simulink model "limited_bit_width_sum_enob"  (R2013b)
settings: Solver=VariableStepDiscrete  StartTime=0.0  StopTime=StopTime  RelTol=1e-3
values from neighbouring files (symbols this model uses):
  a2 = a(2)    [design_2ord_sc_sigma_delta_adc_20211008.m]    (also in run_limited_bit_width_sum.m; run_limited_bit_width_sum_enob.m; run_tst1.m)
  amp = umax    [design_2ord_sc_sigma_delta_adc_20211008.m]    (also in run_limited_bit_width_sum.m; run_limited_bit_width_sum_enob.m = 0.8; run_tst1.m = 0.01)
  b1 = b(1)    [design_2ord_sc_sigma_delta_adc_20211008.m]    (also in run_limited_bit_width_sum.m; run_limited_bit_width_sum_enob.m; run_tst1.m)
  c1 = c(1)    [design_2ord_sc_sigma_delta_adc_20211008.m]    (also in run_limited_bit_width_sum.m; run_limited_bit_width_sum_enob.m; run_tst1.m)
  den = 2^(cic_order*log(osr)/log(2))    [design_2ord_sc_sigma_delta_adc_20211008.m]    (also in run_limited_bit_width_sum.m; run_limited_bit_width_sum_enob.m; run_tst1.m)
  fin = fs*7/128/osr    (= 0.213623046875)    [design_2ord_sc_sigma_delta_adc_20211008.m]    (also in run_limited_bit_width_sum.m = 54.6875; run_limited_bit_width_sum_enob.m; run_tst1.m = 54.6875)
  fs = 256e3    (= 256000)    [design_2ord_sc_sigma_delta_adc_20211008.m]    (also in run_limited_bit_width_sum.m; run_limited_bit_width_sum_enob.m; run_tst1.m)
  osr = 2^16    (= 65536)    [cal_c1_20211015.m]    (also in design_2ord_sc_sigma_delta_adc_20211008.m; run_limited_bit_width_sum.m = 256; run_limited_bit_width_sum_enob.m; run_tst1.m = 256)
  vos = 10e-3    (= 0.01)    [design_2ord_sc_sigma_delta_adc_20211008.m]    (also in run_limited_bit_width_sum.m; run_limited_bit_width_sum_enob.m)
  width_comb1 = 25    [design_2ord_sc_sigma_delta_adc_20211008.m]    (also in run_limited_bit_width_sum.m = width_comb1 - 1; run_limited_bit_width_sum_enob.m = width_comb1 + 1)
  width_comb2 = 20    [design_2ord_sc_sigma_delta_adc_20211008.m]    (also in run_limited_bit_width_sum.m = width_comb2 - 1; run_limited_bit_width_sum_enob.m = width_comb2 + 1)
  width_comb3 = 19    [design_2ord_sc_sigma_delta_adc_20211008.m]    (also in run_limited_bit_width_sum.m = width_comb3 - 1; run_limited_bit_width_sum_enob.m = width_comb3 + 1)
  width_int1 = 49    [design_2ord_sc_sigma_delta_adc_20211008.m]    (also in run_limited_bit_width_sum.m = width_int1 - 1; run_limited_bit_width_sum_enob.m = width_int1 + 1)
  width_int2 = 38    [design_2ord_sc_sigma_delta_adc_20211008.m]    (also in run_limited_bit_width_sum.m = width_int2 - 1; run_limited_bit_width_sum_enob.m = width_int2 + 1)
  width_int3 = 26    [design_2ord_sc_sigma_delta_adc_20211008.m]    (also in run_limited_bit_width_sum.m = width_int3 - 1; run_limited_bit_width_sum_enob.m = width_int3 + 1)
settings Model: Creator=eric  LastModifiedBy=eric

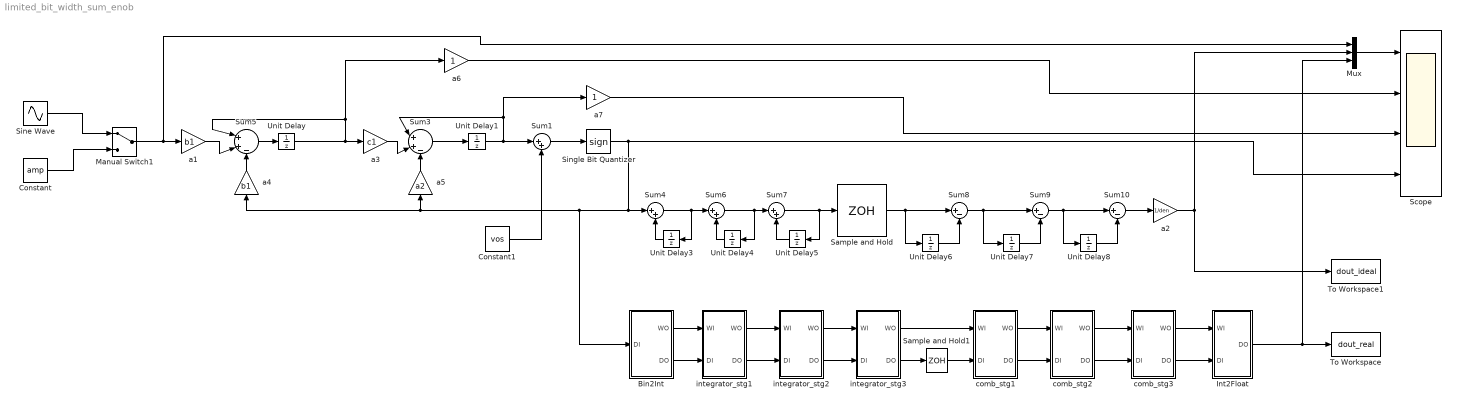
== system limited_bit_width_sum_enob ==
  Bin2Int : Subsystem
  Constant : Constant  Value=amp  SampleTime=1/fs
  Constant1 : Constant  Value=vos  SampleTime=1/fs
  Int2Float : Subsystem
  Manual Switch1 : ManualSwitch
  Mux : Mux  Inputs=3
  Sample and Hold : ZeroOrderHold  SampleTime=osr/fs
  Sample and Hold1 : ZeroOrderHold  SampleTime=osr/fs
  Scope : Scope  NumInputPorts=4
      settings: TimeRange=0.09  YMin=0.00999~-0.2~-0.2~-1.5  YMax=0.01001~0.6~0.2~1.5  MaxDataPoints=20000
  Sine Wave : Sin  Amplitude=amp  Frequency=2*pi*fin  SampleTime=1/fs
  Single Bit Quantizer : Signum  SampleTime=1/fs
  Sum{1,4,6..7} (4 alike) : Sum  Inputs=|++  AccumDataTypeStr=double  SampleTime=1/fs
  Sum10 : Sum  Inputs=|+-  AccumDataTypeStr=double  SampleTime=osr/fs
  Sum3 : Sum  Inputs=|++-  AccumDataTypeStr=double  SampleTime=1/fs
  Sum5 : Sum  Inputs=|++-  AccumDataTypeStr=double  SampleTime=1/fs
  Sum8 : Sum  Inputs=|+-  AccumDataTypeStr=double  SampleTime=osr/fs
  Sum9 : Sum  Inputs=|+-  AccumDataTypeStr=double  SampleTime=osr/fs
  To Workspace : ToWorkspace  VariableName=dout_real  SampleTime=osr/fs  SaveFormat=Timeseries
  To Workspace1 : ToWorkspace  VariableName=dout_ideal  SampleTime=osr/fs  SaveFormat=Timeseries
  Unit Delay{,1,3..5} (5 alike) : UnitDelay  SampleTime=1/fs
  Unit Delay6 : UnitDelay  SampleTime=osr/fs
  Unit Delay7 : UnitDelay  SampleTime=osr/fs
  Unit Delay8 : UnitDelay  SampleTime=osr/fs
  a1 : Gain  Gain=b1  SampleTime=1/fs
  a2 : Gain  Gain=1/den  SampleTime=osr/fs
  a3 : Gain  Gain=c1  SampleTime=1/fs
  a4 : Gain  Gain=b1  SampleTime=1/fs
  a5 : Gain  Gain=a2  SampleTime=1/fs
  a6 : Gain  SampleTime=1/fs
  a7 : Gain  SampleTime=1/fs
  comb_stg1 : Subsystem
  comb_stg2 : Subsystem
  comb_stg3 : Subsystem
  integrator_stg1 : Subsystem
  integrator_stg2 : Subsystem
  integrator_stg3 : Subsystem
  wires:
  Sum3/1 -> Unit Delay1/1
  Sum5/1 -> Unit Delay/1
  Unit Delay3/1 -> Sum4/2
  Sum4/1 -> Sum6/1, Unit Delay3/1
  Unit Delay4/1 -> Sum6/2
  Sum6/1 -> Unit Delay4/1, Sum7/1
  Unit Delay5/1 -> Sum7/2
  Sum7/1 -> Unit Delay5/1, Sample and Hold/1
  Sample and Hold/1 -> Unit Delay6/1, Sum8/1
  Unit Delay6/1 -> Sum8/2
  Unit Delay7/1 -> Sum9/2
  Sum8/1 -> Unit Delay7/1, Sum9/1
  Sum9/1 -> Unit Delay8/1, Sum10/1
  Unit Delay8/1 -> Sum10/2
  Sum10/1 -> a2/1
  a2/1 -> To Workspace1/1, Mux/2
  Manual Switch1/1 -> Mux/1, a1/1
  Sine Wave/1 -> Manual Switch1/1
  Constant/1 -> Manual Switch1/2
  Mux/1 -> Scope/1
  a4/1 -> Sum5/3
  a1/1 -> Sum5/2
  Unit Delay/1 -> a6/1, Sum5/1, a3/1
  a5/1 -> Sum3/3
  a3/1 -> Sum3/2
  Unit Delay1/1 -> Sum1/1, a7/1, Sum3/1
  a7/1 -> Scope/3
  a6/1 -> Scope/2
  Sum1/1 -> Single Bit Quantizer/1
  Constant1/1 -> Sum1/2
  integrator_stg1/1(WO) -> integrator_stg2/1(WI)
  integrator_stg1/2(DO) -> integrator_stg2/2(DI)
  integrator_stg2/1(WO) -> integrator_stg3/1(WI)
  integrator_stg2/2(DO) -> integrator_stg3/2(DI)
  comb_stg1/2(DO) -> comb_stg2/2(DI)
  comb_stg1/1(WO) -> comb_stg2/1(WI)
  comb_stg2/1(WO) -> comb_stg3/1(WI)
  comb_stg2/2(DO) -> comb_stg3/2(DI)
  integrator_stg3/1(WO) -> comb_stg1/1(WI)
  integrator_stg3/2(DO) -> Sample and Hold1/1
  Sample and Hold1/1 -> comb_stg1/2(DI)
  comb_stg3/1(WO) -> Int2Float/1(WI)
  comb_stg3/2(DO) -> Int2Float/2(DI)
  Int2Float/1(DO) -> To Workspace/1, Mux/3
  Single Bit Quantizer/1 -> Bin2Int/1(DI), a5/1, a4/1, Sum4/1, Scope/4
  Bin2Int/1(WO) -> integrator_stg1/1(WI)
  Bin2Int/2(DO) -> integrator_stg1/2(DI)

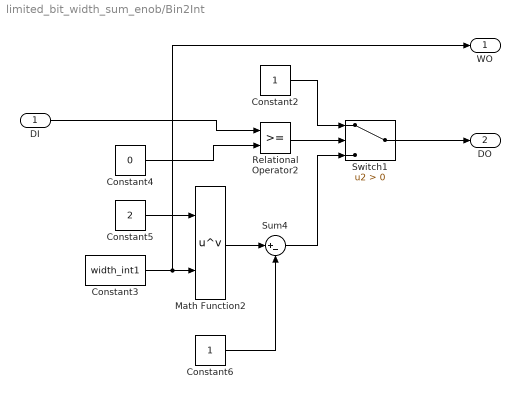
== system limited_bit_width_sum_enob/Bin2Int ==
  DI : Inport
  Constant2 : Constant
  Constant3 : Constant  Value=width_int1
  Constant4 : Constant  Value=0
  Constant5 : Constant  Value=2
  Constant6 : Constant
  Math Function2 : Math  Operator=pow  SampleTime=1/fs  SaturateOnIntegerOverflow=on
  Relational Operator2 : RelationalOperator  OutDataTypeStr=boolean  SampleTime=1/fs
  Sum4 : Sum  Inputs=|+-  SampleTime=1/fs
  Switch1 : Switch  Criteria=u2 > Threshold  SampleTime=1/fs
  WO : Outport
  DO : Outport  Port=2
  wires:
  Math Function2/1 -> Sum4/1
  Constant3/1 -> WO/1, Math Function2/2
  DI/1 -> Relational Operator2/1
  Switch1/1 -> DO/1
  Constant6/1 -> Sum4/2
  Relational Operator2/1 -> Switch1/2
  Constant2/1 -> Switch1/1
  Constant4/1 -> Relational Operator2/2
  Constant5/1 -> Math Function2/1
  Sum4/1 -> Switch1/3

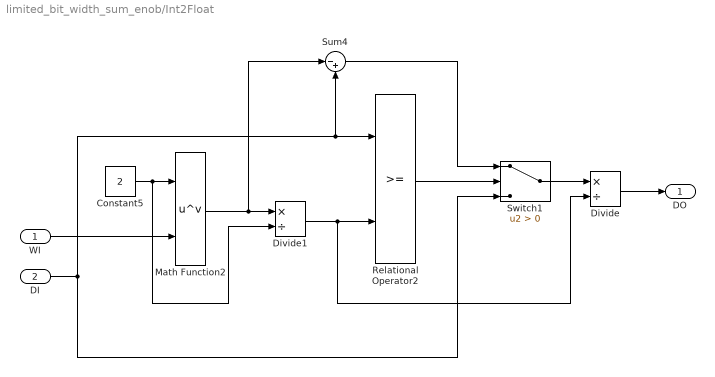
== system limited_bit_width_sum_enob/Int2Float ==
  WI : Inport
  DI : Inport  Port=2
  Constant5 : Constant  Value=2
  Divide : Product  Inputs=*/  SampleTime=1/fs
  Divide1 : Product  Inputs=*/  SampleTime=1/fs
  Math Function2 : Math  Operator=pow  SampleTime=1/fs  SaturateOnIntegerOverflow=on
  Relational Operator2 : RelationalOperator  OutDataTypeStr=boolean  SampleTime=1/fs
  Sum4 : Sum  Inputs=|-+  SampleTime=1/fs
  Switch1 : Switch  Criteria=u2 > Threshold  SampleTime=1/fs
  DO : Outport
  wires:
  Switch1/1 -> Divide/1
  Divide/1 -> DO/1
  Relational Operator2/1 -> Switch1/2
  Math Function2/1 -> Divide1/1, Sum4/1
  Sum4/1 -> Switch1/1
  Constant5/1 -> Divide1/2, Math Function2/1
  DI/1 -> Relational Operator2/1, Sum4/2, Switch1/3
  WI/1 -> Math Function2/2
  Divide1/1 -> Divide/2, Relational Operator2/2

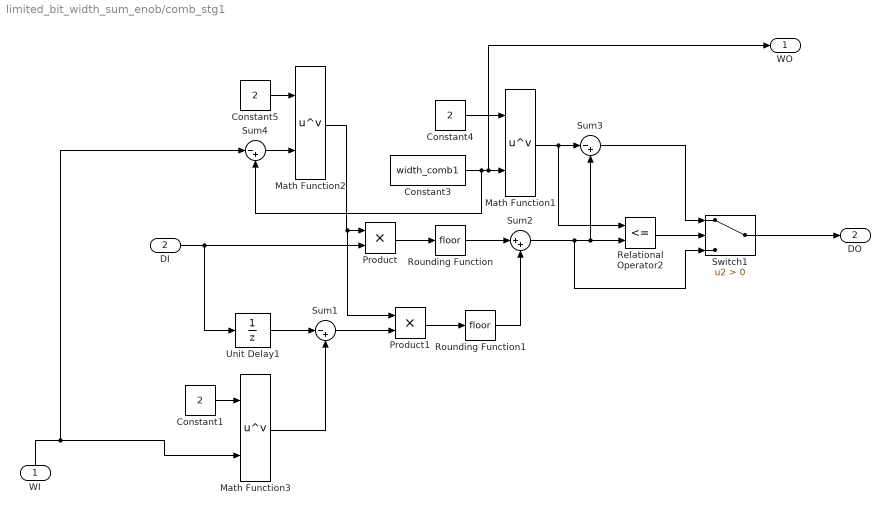
== system limited_bit_width_sum_enob/comb_stg1 ==
  WI : Inport
  DI : Inport  Port=2
  Constant1 : Constant  Value=2
  Constant3 : Constant  Value=width_comb1
  Constant4 : Constant  Value=2
  Constant5 : Constant  Value=2
  Math Function1 : Math  Operator=pow  SampleTime=1/fs  SaturateOnIntegerOverflow=on
  Math Function2 : Math  Operator=pow  SampleTime=1/fs  SaturateOnIntegerOverflow=on
  Math Function3 : Math  Operator=pow  SampleTime=1/fs  SaturateOnIntegerOverflow=on
  Product : Product  SampleTime=1/fs
  Product1 : Product  SampleTime=1/fs
  Relational Operator2 : RelationalOperator  Operator=<=  OutDataTypeStr=boolean  SampleTime=1/fs
  Rounding Function : Rounding  SampleTime=1/fs
  Rounding Function1 : Rounding  SampleTime=1/fs
  Sum1 : Sum  Inputs=|-+  SampleTime=1/fs
  Sum2 : Sum  Inputs=|++  SampleTime=1/fs
  Sum3 : Sum  Inputs=|-+  SampleTime=1/fs
  Sum4 : Sum  Inputs=|-+  SampleTime=1/fs
  Switch1 : Switch  Criteria=u2 > Threshold  SampleTime=1/fs
  Unit Delay1 : UnitDelay  SampleTime=osr/fs
  WO : Outport
  DO : Outport  Port=2
  wires:
  Sum4/1 -> Math Function2/2
  Constant5/1 -> Math Function2/1
  Rounding Function/1 -> Sum2/1
  Math Function2/1 -> Product1/1, Product/1
  Math Function1/1 -> Relational Operator2/1, Sum3/1
  Relational Operator2/1 -> Switch1/2
  Sum3/1 -> Switch1/1
  Sum2/1 -> Relational Operator2/2, Sum3/2, Switch1/3
  Product/1 -> Rounding Function/1
  Constant4/1 -> Math Function1/1
  WI/1 -> Math Function3/2, Sum4/1
  DI/1 -> Unit Delay1/1, Product/2
  Switch1/1 -> DO/1
  Constant1/1 -> Math Function3/1
  Constant3/1 -> Sum4/2, WO/1, Math Function1/2
  Unit Delay1/1 -> Sum1/1
  Math Function3/1 -> Sum1/2
  Rounding Function1/1 -> Sum2/2
  Product1/1 -> Rounding Function1/1
  Sum1/1 -> Product1/2

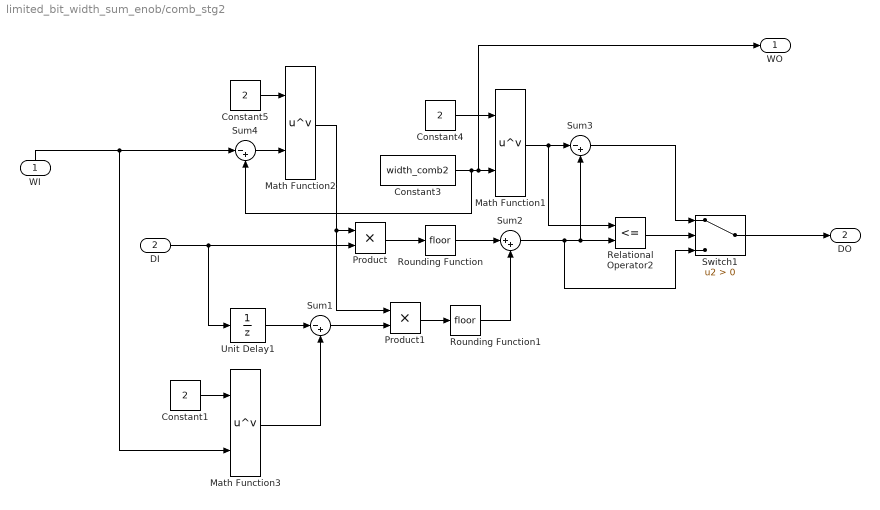
== system limited_bit_width_sum_enob/comb_stg2 ==
  WI : Inport
  DI : Inport  Port=2
  Constant1 : Constant  Value=2
  Constant3 : Constant  Value=width_comb2
  Constant4 : Constant  Value=2
  Constant5 : Constant  Value=2
  Math Function1 : Math  Operator=pow  SampleTime=1/fs  SaturateOnIntegerOverflow=on
  Math Function2 : Math  Operator=pow  SampleTime=1/fs  SaturateOnIntegerOverflow=on
  Math Function3 : Math  Operator=pow  SampleTime=1/fs  SaturateOnIntegerOverflow=on
  Product : Product  SampleTime=1/fs
  Product1 : Product  SampleTime=1/fs
  Relational Operator2 : RelationalOperator  Operator=<=  OutDataTypeStr=boolean  SampleTime=1/fs
  Rounding Function : Rounding  SampleTime=1/fs
  Rounding Function1 : Rounding  SampleTime=1/fs
  Sum1 : Sum  Inputs=|-+  SampleTime=1/fs
  Sum2 : Sum  Inputs=|++  SampleTime=1/fs
  Sum3 : Sum  Inputs=|-+  SampleTime=1/fs
  Sum4 : Sum  Inputs=|-+  SampleTime=1/fs
  Switch1 : Switch  Criteria=u2 > Threshold  SampleTime=1/fs
  Unit Delay1 : UnitDelay  SampleTime=osr/fs
  WO : Outport
  DO : Outport  Port=2
  wires:
  Sum4/1 -> Math Function2/2
  Constant5/1 -> Math Function2/1
  Rounding Function/1 -> Sum2/1
  Math Function2/1 -> Product1/1, Product/1
  Math Function1/1 -> Relational Operator2/1, Sum3/1
  Relational Operator2/1 -> Switch1/2
  Sum3/1 -> Switch1/1
  Sum2/1 -> Relational Operator2/2, Sum3/2, Switch1/3
  Product/1 -> Rounding Function/1
  Constant4/1 -> Math Function1/1
  WI/1 -> Math Function3/2, Sum4/1
  DI/1 -> Unit Delay1/1, Product/2
  Switch1/1 -> DO/1
  Constant1/1 -> Math Function3/1
  Constant3/1 -> Sum4/2, WO/1, Math Function1/2
  Unit Delay1/1 -> Sum1/1
  Math Function3/1 -> Sum1/2
  Rounding Function1/1 -> Sum2/2
  Product1/1 -> Rounding Function1/1
  Sum1/1 -> Product1/2

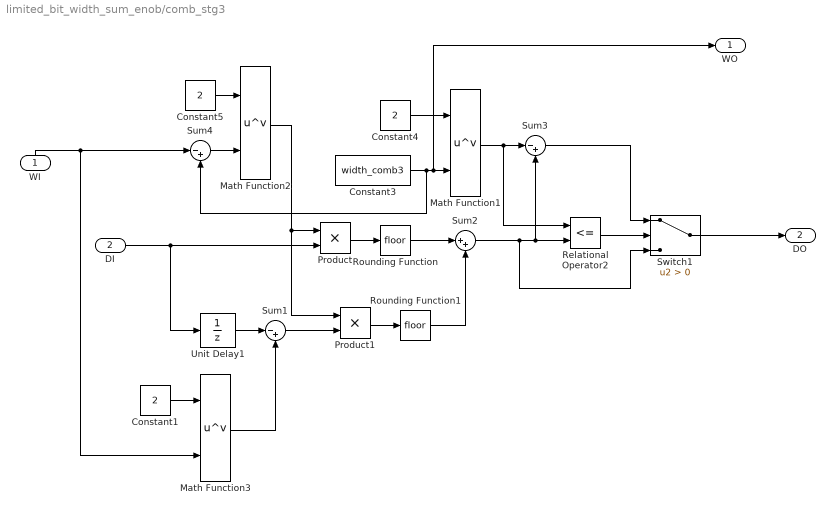
== system limited_bit_width_sum_enob/comb_stg3 ==
  WI : Inport
  DI : Inport  Port=2
  Constant1 : Constant  Value=2
  Constant3 : Constant  Value=width_comb3
  Constant4 : Constant  Value=2
  Constant5 : Constant  Value=2
  Math Function1 : Math  Operator=pow  SampleTime=1/fs  SaturateOnIntegerOverflow=on
  Math Function2 : Math  Operator=pow  SampleTime=1/fs  SaturateOnIntegerOverflow=on
  Math Function3 : Math  Operator=pow  SampleTime=1/fs  SaturateOnIntegerOverflow=on
  Product : Product  SampleTime=1/fs
  Product1 : Product  SampleTime=1/fs
  Relational Operator2 : RelationalOperator  Operator=<=  OutDataTypeStr=boolean  SampleTime=1/fs
  Rounding Function : Rounding  SampleTime=1/fs
  Rounding Function1 : Rounding  SampleTime=1/fs
  Sum1 : Sum  Inputs=|-+  SampleTime=1/fs
  Sum2 : Sum  Inputs=|++  SampleTime=1/fs
  Sum3 : Sum  Inputs=|-+  SampleTime=1/fs
  Sum4 : Sum  Inputs=|-+  SampleTime=1/fs
  Switch1 : Switch  Criteria=u2 > Threshold  SampleTime=1/fs
  Unit Delay1 : UnitDelay  SampleTime=osr/fs
  WO : Outport
  DO : Outport  Port=2
  wires:
  Sum4/1 -> Math Function2/2
  Constant5/1 -> Math Function2/1
  Rounding Function/1 -> Sum2/1
  Math Function2/1 -> Product1/1, Product/1
  Math Function1/1 -> Relational Operator2/1, Sum3/1
  Relational Operator2/1 -> Switch1/2
  Sum3/1 -> Switch1/1
  Sum2/1 -> Relational Operator2/2, Sum3/2, Switch1/3
  Product/1 -> Rounding Function/1
  Constant4/1 -> Math Function1/1
  WI/1 -> Sum4/1, Math Function3/2
  Switch1/1 -> DO/1
  Constant1/1 -> Math Function3/1
  Constant3/1 -> Sum4/2, WO/1, Math Function1/2
  Unit Delay1/1 -> Sum1/1
  Math Function3/1 -> Sum1/2
  DI/1 -> Unit Delay1/1, Product/2
  Product1/1 -> Rounding Function1/1
  Rounding Function1/1 -> Sum2/2
  Sum1/1 -> Product1/2

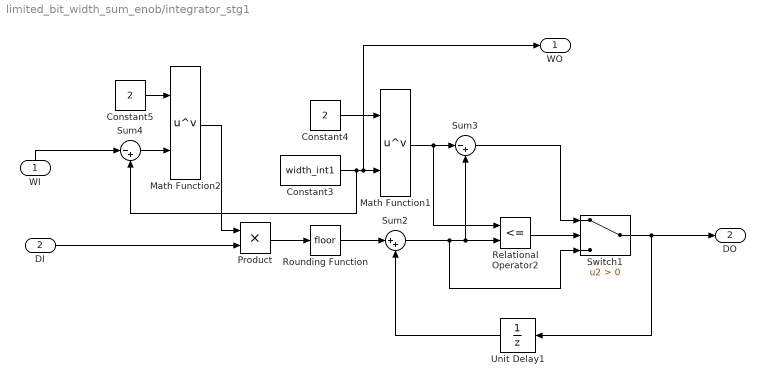
== system limited_bit_width_sum_enob/integrator_stg1 ==
  WI : Inport
  DI : Inport  Port=2
  Constant3 : Constant  Value=width_int1
  Constant4 : Constant  Value=2
  Constant5 : Constant  Value=2
  Math Function1 : Math  Operator=pow  SampleTime=1/fs  SaturateOnIntegerOverflow=on
  Math Function2 : Math  Operator=pow  SampleTime=1/fs  SaturateOnIntegerOverflow=on
  Product : Product  SampleTime=1/fs
  Relational Operator2 : RelationalOperator  Operator=<=  OutDataTypeStr=boolean  SampleTime=1/fs
  Rounding Function : Rounding  SampleTime=1/fs
  Sum2 : Sum  Inputs=|++  SampleTime=1/fs
  Sum3 : Sum  Inputs=|-+  SampleTime=1/fs
  Sum4 : Sum  Inputs=|-+  SampleTime=1/fs
  Switch1 : Switch  Criteria=u2 > Threshold  SampleTime=1/fs
  Unit Delay1 : UnitDelay  SampleTime=1/fs
  WO : Outport
  DO : Outport  Port=2
  wires:
  Sum4/1 -> Math Function2/2
  Constant5/1 -> Math Function2/1
  Rounding Function/1 -> Sum2/1
  Math Function2/1 -> Product/1
  Math Function1/1 -> Relational Operator2/1, Sum3/1
  Relational Operator2/1 -> Switch1/2
  Sum3/1 -> Switch1/1
  Sum2/1 -> Relational Operator2/2, Sum3/2, Switch1/3
  Product/1 -> Rounding Function/1
  Constant4/1 -> Math Function1/1
  Unit Delay1/1 -> Sum2/2
  WI/1 -> Sum4/1
  DI/1 -> Product/2
  Constant3/1 -> Sum4/2, WO/1, Math Function1/2
  Switch1/1 -> Unit Delay1/1, DO/1

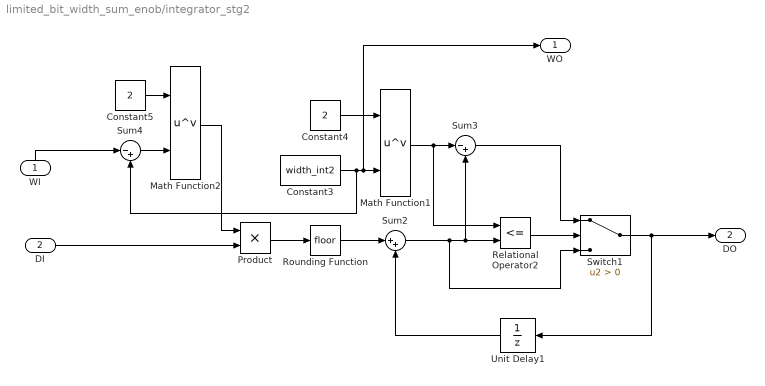
== system limited_bit_width_sum_enob/integrator_stg2 ==
  WI : Inport
  DI : Inport  Port=2
  Constant3 : Constant  Value=width_int2
  Constant4 : Constant  Value=2
  Constant5 : Constant  Value=2
  Math Function1 : Math  Operator=pow  SampleTime=1/fs  SaturateOnIntegerOverflow=on
  Math Function2 : Math  Operator=pow  SampleTime=1/fs  SaturateOnIntegerOverflow=on
  Product : Product  SampleTime=1/fs
  Relational Operator2 : RelationalOperator  Operator=<=  OutDataTypeStr=boolean  SampleTime=1/fs
  Rounding Function : Rounding  SampleTime=1/fs
  Sum2 : Sum  Inputs=|++  SampleTime=1/fs
  Sum3 : Sum  Inputs=|-+  SampleTime=1/fs
  Sum4 : Sum  Inputs=|-+  SampleTime=1/fs
  Switch1 : Switch  Criteria=u2 > Threshold  SampleTime=1/fs
  Unit Delay1 : UnitDelay  SampleTime=1/fs
  WO : Outport
  DO : Outport  Port=2
  wires:
  Sum4/1 -> Math Function2/2
  Constant5/1 -> Math Function2/1
  Rounding Function/1 -> Sum2/1
  Math Function2/1 -> Product/1
  Math Function1/1 -> Relational Operator2/1, Sum3/1
  Relational Operator2/1 -> Switch1/2
  Sum3/1 -> Switch1/1
  Sum2/1 -> Relational Operator2/2, Sum3/2, Switch1/3
  Product/1 -> Rounding Function/1
  Constant4/1 -> Math Function1/1
  Unit Delay1/1 -> Sum2/2
  WI/1 -> Sum4/1
  DI/1 -> Product/2
  Constant3/1 -> Sum4/2, WO/1, Math Function1/2
  Switch1/1 -> Unit Delay1/1, DO/1

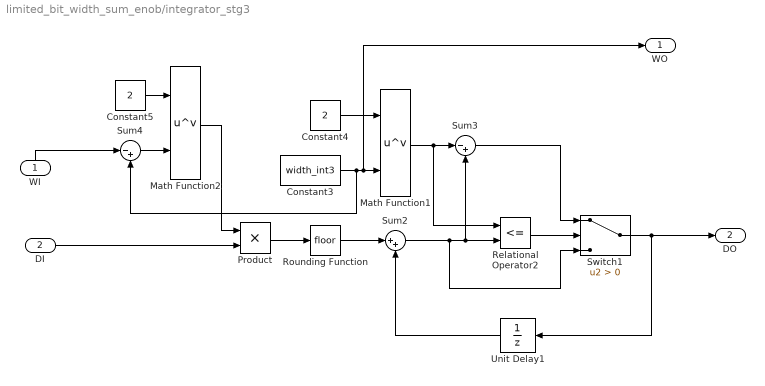
== system limited_bit_width_sum_enob/integrator_stg3 ==
  WI : Inport
  DI : Inport  Port=2
  Constant3 : Constant  Value=width_int3
  Constant4 : Constant  Value=2
  Constant5 : Constant  Value=2
  Math Function1 : Math  Operator=pow  SampleTime=1/fs  SaturateOnIntegerOverflow=on
  Math Function2 : Math  Operator=pow  SampleTime=1/fs  SaturateOnIntegerOverflow=on
  Product : Product  SampleTime=1/fs
  Relational Operator2 : RelationalOperator  Operator=<=  OutDataTypeStr=boolean  SampleTime=1/fs
  Rounding Function : Rounding  SampleTime=1/fs
  Sum2 : Sum  Inputs=|++  SampleTime=1/fs
  Sum3 : Sum  Inputs=|-+  SampleTime=1/fs
  Sum4 : Sum  Inputs=|-+  SampleTime=1/fs
  Switch1 : Switch  Criteria=u2 > Threshold  SampleTime=1/fs
  Unit Delay1 : UnitDelay  SampleTime=1/fs
  WO : Outport
  DO : Outport  Port=2
  wires:
  Sum4/1 -> Math Function2/2
  Constant5/1 -> Math Function2/1
  Rounding Function/1 -> Sum2/1
  Math Function2/1 -> Product/1
  Math Function1/1 -> Relational Operator2/1, Sum3/1
  Relational Operator2/1 -> Switch1/2
  Sum3/1 -> Switch1/1
  Sum2/1 -> Relational Operator2/2, Sum3/2, Switch1/3
  Product/1 -> Rounding Function/1
  Constant4/1 -> Math Function1/1
  Unit Delay1/1 -> Sum2/2
  WI/1 -> Sum4/1
  DI/1 -> Product/2
  Constant3/1 -> Sum4/2, WO/1, Math Function1/2
  Switch1/1 -> Unit Delay1/1, DO/1
